simulink library "SpeedEstimater"  (R2023b)
settings: Solver=VariableStepAuto  StartTime=0.0  StopTime=10.0  RelTol=1e-3
libraries: arduinolib x2, simulink x1, hdlsllib_double x1
settings Model: Creator=user  LastModifiedBy=user

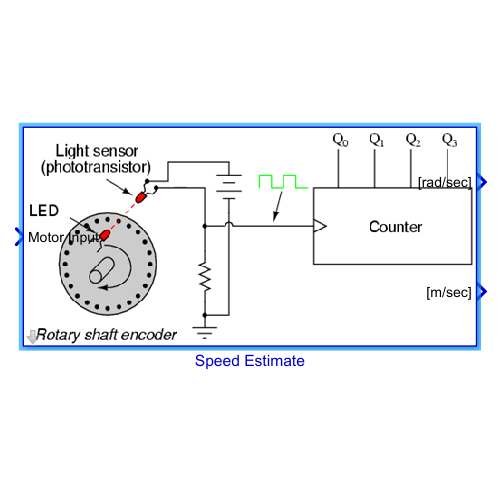
[thumbnail: Simulink's stored preview of the top-level diagram]
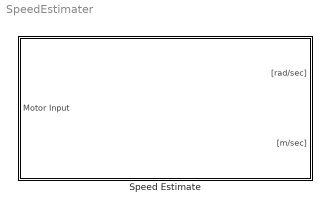
== system SpeedEstimater ==
  Speed Estimate : Subsystem  mask{pinExt=2, pinA=4, r=0.032, Ts=-1, pulse=1560}
      mask prompts: pinExt "外部割込み信号 Pin："; pinA "エンコーダ APin："; r "タイヤ半径 r [m]："; Ts "サンプリング周期 Ts [m]："; pulse "モータが1回転するときのパルス数："
      mask TypeOptions pinExt: External Interrupt/Pin
      mask TypeOptions pinA:
      | Function-Call
      | Subsystem/Digital Input/pinNumber
      mask DialogControl Parameter Prompt: Parameter
      mask Display: image('Encoder.png');

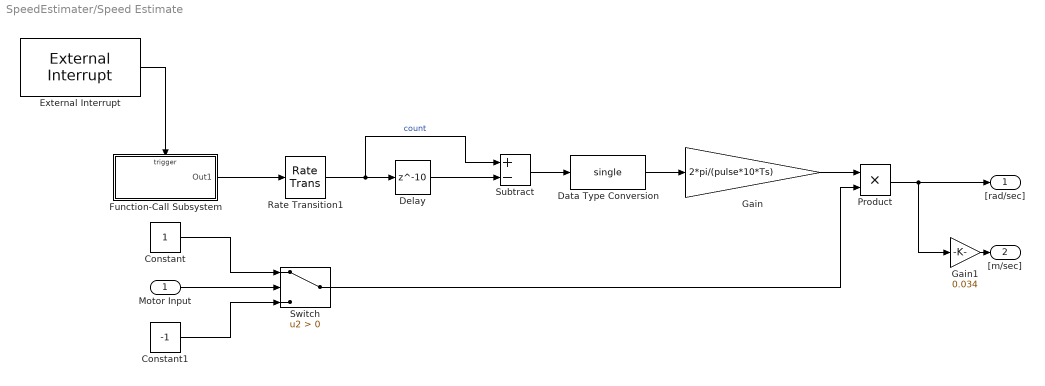
== system SpeedEstimater/Speed Estimate ==
  Motor Input : Inport
  Constant : Constant
  Constant1 : Constant  Value=-1
  Data Type Conversion : DataTypeConversion  OutDataTypeStr=single  SaturateOnIntegerOverflow=off  RndMeth=Floor
  Delay : Delay  DelayLength=10
  External Interrupt : arduinolib/External Interrupt  Pin=pinExt  PullUp=off  Mode=RISING  InterruptSimulationInput=off
  Function-Call Subsystem : Subsystem  TreatAsAtomicUnit=on
  Gain : Gain  Gain=2*pi/(pulse*10*Ts)
  Gain1 : Gain  Gain=0.034
  Product : Product
  Rate Transition1 : RateTransition  Deterministic=off
  Subtract : Sum  Inputs=+-
  Switch : Switch  Criteria=u2 > Threshold  SaturateOnIntegerOverflow=off  InputSameDT=off
  "[rad/sec]" : Outport
  "[m/sec]" : Outport  Port=2
  wires:
  Rate Transition1/1 -> Subtract/1, Delay/1  "count"
  External Interrupt/1 -> Function-Call Subsystem/Trigger
  Function-Call Subsystem/1(Out1) -> Rate Transition1/1
  Delay/1 -> Subtract/2
  Subtract/1 -> Data Type Conversion/1
  Data Type Conversion/1 -> Gain/1
  Gain1/1 -> "[m/sec]"/1
  Motor Input/1 -> Switch/2
  Constant/1 -> Switch/1
  Constant1/1 -> Switch/3
  Product/1 -> "[rad/sec]"/1, Gain1/1
  Gain/1 -> Product/1
  Switch/1 -> Product/2

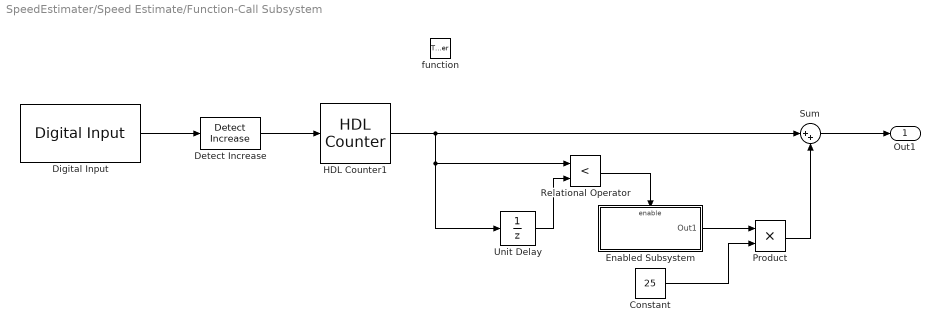
== system SpeedEstimater/Speed Estimate/Function-Call Subsystem ==
  function : TriggerPort  TriggerType=function-call  VariantControl=(inherit)
  Constant : Constant  Value=25
  Detect Increase : simulink/Logic and Bit Operations/Detect Increase  vinit=0.0  OutDataTypeStr=boolean
  Digital Input : arduinolib/Digital Input  pinNumber=pinA  mode=Default  Direction=input  SampleTime=-1  blockPlatform=arduino
  Enabled Subsystem : Subsystem  TreatAsAtomicUnit=on
  HDL Counter1 : hdlsllib_double/Sources/HDL Counter  CountType=Count limited  CountInit=0  CountStep=1  CountMax=25  CountFromType=Initial value  CountFrom=0  CountResetPort=off  CountLoadPort=off  CountEnbPort=on  CountDirPort=off  CountHitOutputPort=off  CountDataType=Signed  CountWordLen=16  CountFracLen=0  CountSampTime=1
  Product : Product
  Relational Operator : RelationalOperator  Operator=<  OutDataTypeStr=boolean  RndMeth=Simplest  InputSameDT=off
  Sum : Sum  Inputs=|++
  Unit Delay : UnitDelay  SampleTime=-1  HasFrameUpgradeWarning=on
  Out1 : Outport
  wires:
  Digital Input/1 -> Detect Increase/1
  Detect Increase/1 -> HDL Counter1/1
  Sum/1 -> Out1/1
  HDL Counter1/1 -> Sum/1, Unit Delay/1, Relational Operator/1
  Enabled Subsystem/1(Out1) -> Product/1
  Product/1 -> Sum/2
  Constant/1 -> Product/2
  Relational Operator/1 -> Enabled Subsystem/Enable
  Unit Delay/1 -> Relational Operator/2

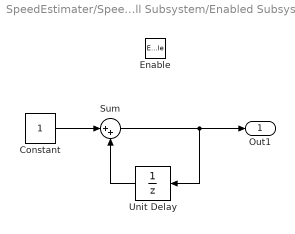
== system SpeedEstimater/Speed Estimate/Function-Call Subsystem/Enabled Subsystem ==
  Enable : EnablePort
  Constant : Constant
  Sum : Sum  Inputs=|++
  Unit Delay : UnitDelay  SampleTime=-1  HasFrameUpgradeWarning=on
  Out1 : Outport
  wires:
  Constant/1 -> Sum/1
  Sum/1 -> Unit Delay/1, Out1/1
  Unit Delay/1 -> Sum/2
